simulink model "LQR_simulation"  (R2021a)
settings: Solver=VariableStepAuto  StartTime=0.0  StopTime=t_final  RelTol=1e-3
values from neighbouring files (symbols this model uses):
  A = [0 1 0 0 ... (first row only)    [Controllability_of_a_Linear_System.m]    (also in Full_State_Feedback_Control_Design.m = [0 3;2 4]; Implementation_Issues_with_a_FSFB.m = [0 1 0; Introduction_to_Full_State_Feedback_COntrol.m = [0 3;2 4]; Introduction_to_LQR_control.m = [0 1)
  B = [0 ... (first row only)    [Controllability_of_a_Linear_System.m]    (also in Full_State_Feedback_Control_Design.m = [-2 1; 1 1]; Implementation_Issues_with_a_FSFB.m = [0 0; Introduction_to_Full_State_Feedback_COntrol.m = [-2 1; 1 1]; Introduction_to_LQR_control.m)
  K = place(A,B(:,1),desired_closed_loop_poles)    [Implementation_Issues_with_a_FSFB.m]    (also in Practical_Implementation_Issues_with_a_FSFB.m)
  x0 = [72*pi/180 ... (first row only)    [Implementation_Issues_with_a_FSFB.m]    (also in Introduction_to_LQR_control.m = [pi; LQR_control.m = [pi)
settings Model: Creator=subhi  LastModifiedBy=subhi

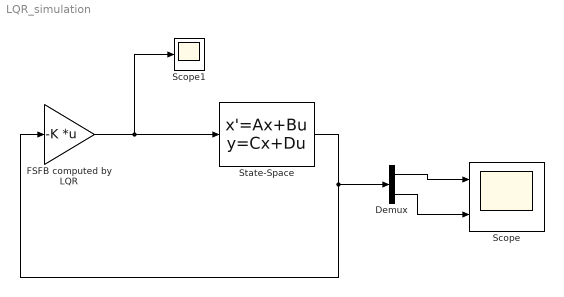
== system LQR_simulation ==
  Demux : Demux  Outputs=2
  FSFB computed by LQR : Gain  Gain=-K  Multiplication=Matrix(K*u)
  Scope : Scope  NumInputPorts=2
  Scope1 : Scope
  State-Space : StateSpace  A=A  B=B  C=eye(2)  D=zeros(2,1)  InitialCondition=x0
  wires:
  FSFB computed by LQR/1 -> Scope1/1, State-Space/1
  State-Space/1 -> FSFB computed by LQR/1, Demux/1
  Demux/1 -> Scope/1
  Demux/2 -> Scope/2
